simulink model "GSandFlare_werkend"  (R2021b)
settings: Solver=VariableStepAuto  StartTime=0.0  StopTime=140  RelTol=1e-3
values from neighbouring files (symbols this model uses):
  A_5 = SS_long_lo.A([1 2 3 4 5],[1 2 3 4 5])    [FindF16Dynamics.m]
  B_5 = SS_long_lo.A([1 2 3 4 5],[6 7])    [FindF16Dynamics.m]
  C_5 = SS_long_lo.C([1 2 3 4 5],[1 2 3 4 5])    [FindF16Dynamics.m]
  D_5 = SS_long_lo.D([1 2 3 4 5],[1 2])    [FindF16Dynamics.m]
  h_airport = 3000    [FindF16Dynamics.m]
  h_flare = x2*tan(GS_angle*(pi/180))    [FindF16Dynamics.m]
  runway_distance = 10*velocity + (2000/tan(GS_angle))    [FindF16Dynamics.m]
  tau = -h_flare/h_dot    [FindF16Dynamics.m]
  trim_alt = altitude    (= 5000)    [FindF16Dynamics.m]
  trim_velocity = velocity    (= 300)    [FindF16Dynamics.m]
undefined symbols (not defined in the file or in its folder): trim_state_lo, trim_thrust_lo
libraries: slpidlib x3
settings Model: Creator=Victor  LastModifiedBy=Victor

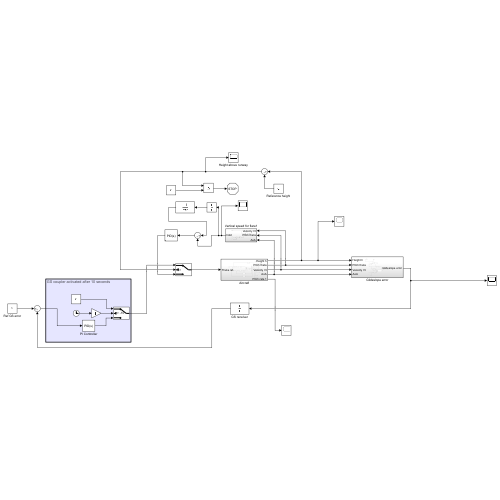
[thumbnail: Simulink's stored preview of the top-level diagram]
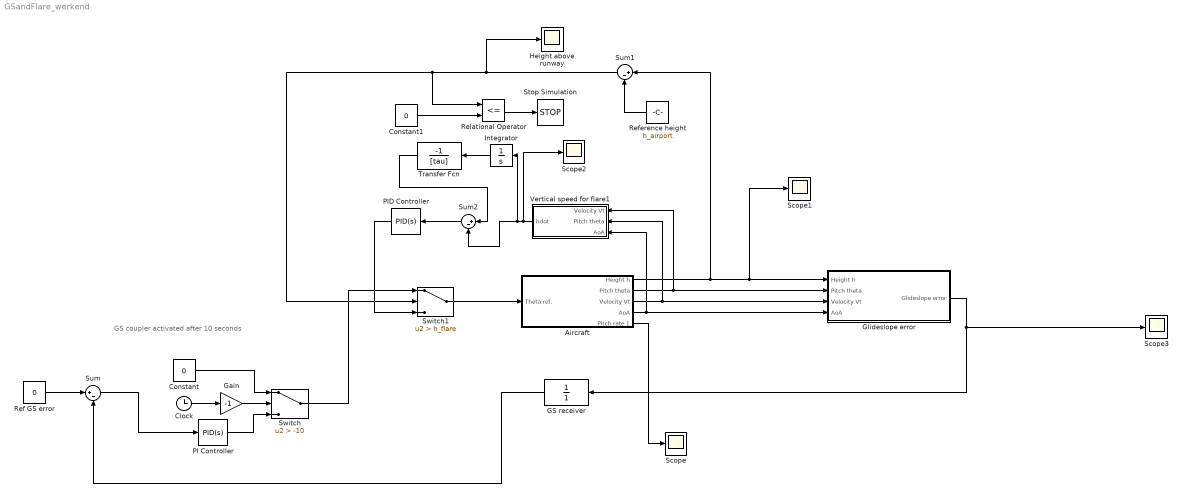
== system GSandFlare_werkend ==
  note: GS coupler activated after 10 seconds
  Aircraft : Subsystem  Tag=Aircraft
  Clock : Clock
  Constant : Constant  Value=0
  Constant1 : Constant  Value=0
  GS receiver : TransferFcn  Denominator=[1]
  Gain : Gain  Gain=-1
  Glideslope error : Subsystem
  Height above runway : Scope
  Integrator : Integrator
  PI Controller : slpidlib/PID Controller  Controller=PID  Form=Parallel  TimeDomain=Continuous-time  UseExternalTs=off  SampleTime=-1  IntegratorMethod=Forward Euler  FilterMethod=Forward Euler  ControllerParametersSource=internal  P=10  I=0.1  D=0  UseFilter=on  N=100  TunerSelectOption=Transfer Function Based (PID Tuner App)  InitialConditionSource=internal  InitialConditionForIntegrator=0  InitialConditionForFilter=0  DifferentiatorICPrevScaledInput=0  ExternalReset=none  TrackingMode=off  Kt=1  LimitOutput=off  SatLimitsSource=internal  UpperSaturationLimit=inf  LowerSaturationLimit=-inf  LinearizeAsGain=on  AntiWindupMode=none  Kb=1  POutMin=[]  POutMax=[]  IOutMin=[]  IOutMax=[]  DOutMin=[]  DOutMax=[]  NOutMin=[]  NOutMax=[]  SumOutMin=[]  SumOutMax=[]  SaturationOutMin=[]  SaturationOutMax=[]  PParamMin=[]  PParamMax=[]  IParamMin=[]  IParamMax=[]  DParamMin=[]  DParamMax=[]  NParamMin=[]  NParamMax=[]  KbParamMin=[]  KbParamMax=[]  KtParamMin=[]  KtParamMax=[]  KbOutMin=[]  KbOutMax=[]  KtOutMin=[]  KtOutMax=[]  IntegratorOutMin=[]  IntegratorOutMax=[]  FilterOutMin=[]  FilterOutMax=[]  SumI1OutMin=[]  SumI1OutMax=[]  SumI2OutMin=[]  SumI2OutMax=[]  SumI3OutMin=[]  SumI3OutMax=[]  SumI4OutMin=[]  SumI4OutMax=[]  SumDOutMin=[]  SumDOutMax=[]  DifferentiatorOutMin=[]  DifferentiatorOutMax=[]  FilterDiffOutCoefMin=[]  FilterDiffOutCoefMax=[]  ReciprocalOutMin=[]  ReciprocalOutMax=[]  SumDenOutMin=[]  SumDenOutMax=[]  SumNumOutMin=[]  SumNumOutMax=[]  DivideOutMin=[]  DivideOutMax=[]  UdiffTsProdOutMin=[]  UdiffTsProdOutMax=[]  NTsProdOutMin=[]  NTsProdOutMax=[]  UintegralTsProdOutMin=[]  UintegralTsProdOutMax=[]  UngainTsProdOutMin=[]  UngainTsProdOutMax=[]  IntegratorContinuousStateAttributes=''  IntegratorStateMustResolveToSignalObject=off  IntegratorRTWStateStorageClass=Auto  FilterContinuousStateAttributes=''  FilterStateMustResolveToSignalObject=off  FilterRTWStateStorageClass=Auto  ParallelPVariant=InternalParameters  IdealPVariant=Disabled  IVariant=InternalParameters  DVariant=InternalParameters  IntegratorVariant=Continuous  SatVariant=Disabled  AWVariant=Passthrough  PCopyVariant=Disabled  TRVariant=Disabled  FdbkBlocksVariant=Forward  IdealPFdbkVariant=Disabled  SatFdbkVariant=Disabled  DerivativeFilterVariant=ContFilter  NVariant=InternalParameters  NCopyVariant=Disabled  FilterICVariant=InternalICsFilter  IntegratorICVariant=InternalICs  ExternalResetVariant=Disabled  TRSumVariant=Passthrough  SumFdbkVariant=Disabled  SumVariant=Sum_PID  TsampFilterVariant=InternalTs  TsampNgainVariant=Passthrough  TsampIntegralVariant=Passthrough  ExternalSaturationOutDataTypeStr=Inherit: Same as second input
  PID Controller : slpidlib/PID Controller  Controller=PID  Form=Parallel  TimeDomain=Continuous-time  UseExternalTs=off  SampleTime=-1  IntegratorMethod=Forward Euler  FilterMethod=Forward Euler  ControllerParametersSource=internal  P=0.001  I=0.0000000001  D=0.45  UseFilter=on  N=100  TunerSelectOption=Transfer Function Based (PID Tuner App)  InitialConditionSource=internal  InitialConditionForIntegrator=0  InitialConditionForFilter=0  DifferentiatorICPrevScaledInput=0  ExternalReset=none  TrackingMode=off  Kt=1  LimitOutput=off  SatLimitsSource=internal  UpperSaturationLimit=inf  LowerSaturationLimit=-inf  LinearizeAsGain=on  AntiWindupMode=none  Kb=1  POutMin=[]  POutMax=[]  IOutMin=[]  IOutMax=[]  DOutMin=[]  DOutMax=[]  NOutMin=[]  NOutMax=[]  SumOutMin=[]  SumOutMax=[]  SaturationOutMin=[]  SaturationOutMax=[]  PParamMin=[]  PParamMax=[]  IParamMin=[]  IParamMax=[]  DParamMin=[]  DParamMax=[]  NParamMin=[]  NParamMax=[]  KbParamMin=[]  KbParamMax=[]  KtParamMin=[]  KtParamMax=[]  KbOutMin=[]  KbOutMax=[]  KtOutMin=[]  KtOutMax=[]  IntegratorOutMin=[]  IntegratorOutMax=[]  FilterOutMin=[]  FilterOutMax=[]  SumI1OutMin=[]  SumI1OutMax=[]  SumI2OutMin=[]  SumI2OutMax=[]  SumI3OutMin=[]  SumI3OutMax=[]  SumI4OutMin=[]  SumI4OutMax=[]  SumDOutMin=[]  SumDOutMax=[]  DifferentiatorOutMin=[]  DifferentiatorOutMax=[]  FilterDiffOutCoefMin=[]  FilterDiffOutCoefMax=[]  ReciprocalOutMin=[]  ReciprocalOutMax=[]  SumDenOutMin=[]  SumDenOutMax=[]  SumNumOutMin=[]  SumNumOutMax=[]  DivideOutMin=[]  DivideOutMax=[]  UdiffTsProdOutMin=[]  UdiffTsProdOutMax=[]  NTsProdOutMin=[]  NTsProdOutMax=[]  UintegralTsProdOutMin=[]  UintegralTsProdOutMax=[]  UngainTsProdOutMin=[]  UngainTsProdOutMax=[]  IntegratorContinuousStateAttributes=''  IntegratorStateMustResolveToSignalObject=off  IntegratorRTWStateStorageClass=Auto  FilterContinuousStateAttributes=''  FilterStateMustResolveToSignalObject=off  FilterRTWStateStorageClass=Auto  ParallelPVariant=InternalParameters  IdealPVariant=Disabled  IVariant=InternalParameters  DVariant=InternalParameters  IntegratorVariant=Continuous  SatVariant=Disabled  AWVariant=Passthrough  PCopyVariant=Disabled  TRVariant=Disabled  FdbkBlocksVariant=Forward  IdealPFdbkVariant=Disabled  SatFdbkVariant=Disabled  DerivativeFilterVariant=ContFilter  NVariant=InternalParameters  NCopyVariant=Disabled  FilterICVariant=InternalICsFilter  IntegratorICVariant=InternalICs  ExternalResetVariant=Disabled  TRSumVariant=Passthrough  SumFdbkVariant=Disabled  SumVariant=Sum_PID  TsampFilterVariant=InternalTs  TsampNgainVariant=Passthrough  TsampIntegralVariant=Passthrough  ExternalSaturationOutDataTypeStr=Inherit: Same as second input
  Ref GS error : Constant  Value=0
  Reference height : Constant  Value=h_airport
  Relational Operator : RelationalOperator  Operator=<=  OutDataTypeStr=boolean  RndMeth=Simplest
  Scope{,1..3} (4 alike) : Scope
  Stop Simulation : Stop
  Sum : Sum  Inputs=|+-
  Sum1 : Sum  Inputs=|+-
  Sum2 : Sum  Inputs=|+-
  Switch : Switch  Criteria=u2 > Threshold  Threshold=-10
  Switch1 : Switch  Criteria=u2 > Threshold  Threshold=h_flare
  Transfer Fcn : TransferFcn  Numerator=[-1]  Denominator=[tau]
  Vertical speed for flare1 : Subsystem
  wires:
  Aircraft/1(Height h) -> Sum1/1, Scope1/1, Glideslope error/1(Height h)
  Aircraft/4(AoA) -> Vertical speed for flare1/3(AoA), Glideslope error/4(AoA)
  Aircraft/2(Pitch theta) -> Vertical speed for flare1/1(Velocity Vt), Glideslope error/2(Pitch theta)
  Glideslope error/1(Glideslope error) -> GS receiver/1, Scope3/1
  Ref GS error/1 -> Sum/1
  GS receiver/1 -> Sum/2
  Sum/1 -> PI Controller/1
  PI Controller/1 -> Switch/3
  Constant/1 -> Switch/1
  Gain/1 -> Switch/2
  Clock/1 -> Gain/1
  Aircraft/3(Velocity Vt) -> Vertical speed for flare1/2(Pitch theta), Glideslope error/3(Velocity Vt)
  Switch/1 -> Switch1/1
  Switch1/1 -> Aircraft/1(Theta ref.)
  Reference height/1 -> Sum1/2
  Sum1/1 -> Height above runway/1, Relational Operator/1, Switch1/2
  Constant1/1 -> Relational Operator/2
  Relational Operator/1 -> Stop Simulation/1
  Aircraft/5(Pitch rate 1) -> Scope/1
  PID Controller/1 -> Switch1/3
  Vertical speed for flare1/1(hdot) -> Scope2/1, Integrator/1, Sum2/2
  Sum2/1 -> PID Controller/1
  Integrator/1 -> Transfer Fcn/1
  Transfer Fcn/1 -> Sum2/1

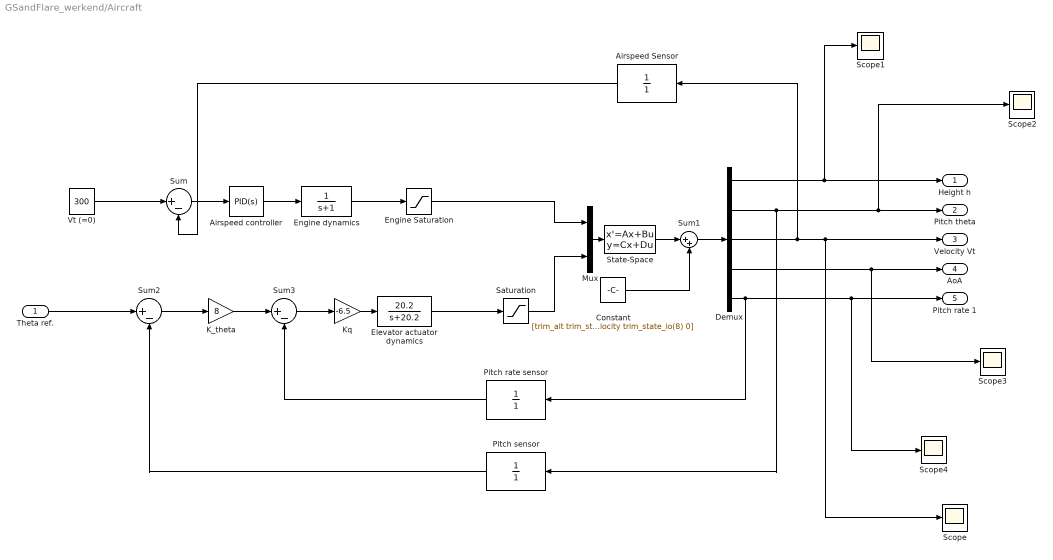
== system GSandFlare_werkend/Aircraft ==
  Theta ref. : Inport
  Airspeed Sensor : TransferFcn  Denominator=[1]
  Airspeed controller : slpidlib/PID Controller  Controller=PID  Form=Parallel  TimeDomain=Continuous-time  UseExternalTs=off  SampleTime=-1  IntegratorMethod=Forward Euler  FilterMethod=Forward Euler  ControllerParametersSource=internal  P=133.541176016203  I=2.35764233778221  D=232.681071797148  UseFilter=on  N=21.8595644116061  TunerSelectOption=Transfer Function Based (PID Tuner App)  InitialConditionSource=internal  InitialConditionForIntegrator=0  InitialConditionForFilter=0  DifferentiatorICPrevScaledInput=0  ExternalReset=none  TrackingMode=off  Kt=1  LimitOutput=off  SatLimitsSource=internal  UpperSaturationLimit=inf  LowerSaturationLimit=-inf  LinearizeAsGain=on  AntiWindupMode=none  Kb=1  POutMin=[]  POutMax=[]  IOutMin=[]  IOutMax=[]  DOutMin=[]  DOutMax=[]  NOutMin=[]  NOutMax=[]  SumOutMin=[]  SumOutMax=[]  SaturationOutMin=[]  SaturationOutMax=[]  PParamMin=[]  PParamMax=[]  IParamMin=[]  IParamMax=[]  DParamMin=[]  DParamMax=[]  NParamMin=[]  NParamMax=[]  KbParamMin=[]  KbParamMax=[]  KtParamMin=[]  KtParamMax=[]  KbOutMin=[]  KbOutMax=[]  KtOutMin=[]  KtOutMax=[]  IntegratorOutMin=[]  IntegratorOutMax=[]  FilterOutMin=[]  FilterOutMax=[]  SumI1OutMin=[]  SumI1OutMax=[]  SumI2OutMin=[]  SumI2OutMax=[]  SumI3OutMin=[]  SumI3OutMax=[]  SumI4OutMin=[]  SumI4OutMax=[]  SumDOutMin=[]  SumDOutMax=[]  DifferentiatorOutMin=[]  DifferentiatorOutMax=[]  FilterDiffOutCoefMin=[]  FilterDiffOutCoefMax=[]  ReciprocalOutMin=[]  ReciprocalOutMax=[]  SumDenOutMin=[]  SumDenOutMax=[]  SumNumOutMin=[]  SumNumOutMax=[]  DivideOutMin=[]  DivideOutMax=[]  UdiffTsProdOutMin=[]  UdiffTsProdOutMax=[]  NTsProdOutMin=[]  NTsProdOutMax=[]  UintegralTsProdOutMin=[]  UintegralTsProdOutMax=[]  UngainTsProdOutMin=[]  UngainTsProdOutMax=[]  IntegratorContinuousStateAttributes=''  IntegratorStateMustResolveToSignalObject=off  IntegratorRTWStateStorageClass=Auto  FilterContinuousStateAttributes=''  FilterStateMustResolveToSignalObject=off  FilterRTWStateStorageClass=Auto  ParallelPVariant=InternalParameters  IdealPVariant=Disabled  IVariant=InternalParameters  DVariant=InternalParameters  IntegratorVariant=Continuous  SatVariant=Disabled  AWVariant=Passthrough  PCopyVariant=Disabled  TRVariant=Disabled  FdbkBlocksVariant=Forward  IdealPFdbkVariant=Disabled  SatFdbkVariant=Disabled  DerivativeFilterVariant=ContFilter  NVariant=InternalParameters  NCopyVariant=Disabled  FilterICVariant=InternalICsFilter  IntegratorICVariant=InternalICs  ExternalResetVariant=Disabled  TRSumVariant=Passthrough  SumFdbkVariant=Disabled  SumVariant=Sum_PID  TsampFilterVariant=InternalTs  TsampNgainVariant=Passthrough  TsampIntegralVariant=Passthrough  ExternalSaturationOutDataTypeStr=Inherit: Same as second input
  Constant : Constant  Value=[trim_alt trim_state_lo(5) trim_velocity trim_state_lo(8) 0]
  Demux : Demux  Outputs=5
  Elevator actuator dynamics : TransferFcn  Numerator=[20.2]  Denominator=[1 20.2]
  Engine Saturation : Saturate  UpperLimit=19000 -trim_thrust_lo  LowerLimit=1000 - trim_thrust_lo
  Engine dynamics : TransferFcn  Denominator=[1 1]
  K_theta : Gain  Gain=8
  Kq : Gain  Gain=-6.5
  Mux : Mux  Inputs=2
  Pitch rate sensor : TransferFcn  Denominator=[1]
  Pitch sensor : TransferFcn  Denominator=[1]
  Saturation : Saturate  UpperLimit=25  LowerLimit=-25
  Scope{,1..4} (5 alike) : Scope
  State-Space : StateSpace  A=A_5  B=B_5  C=C_5  D=D_5  InitialCondition=0  ParameterTunability=Unconstrained
  Sum : Sum  Inputs=|+-
  Sum1 : Sum  Inputs=|++
  Sum2 : Sum  Inputs=|+-
  Sum3 : Sum  Inputs=|+-
  Vt (=0) : Constant  Value=300
  Height h : Outport
  Pitch theta : Outport  Port=2
  Velocity Vt : Outport  Port=3
  AoA : Outport  Port=4
  Pitch rate 1 : Outport  Port=5
  wires:
  Demux/1 -> Scope1/1, Height h/1
  Demux/2 -> Pitch sensor/1, Scope2/1, Pitch theta/1
  Demux/4 -> Scope3/1, AoA/1
  Demux/5 -> Scope4/1, Pitch rate 1/1, Pitch rate sensor/1
  Vt (=0)/1 -> Sum/1
  Airspeed Sensor/1 -> Sum/2
  Sum/1 -> Airspeed controller/1
  Airspeed controller/1 -> Engine dynamics/1
  Engine dynamics/1 -> Engine Saturation/1
  Mux/1 -> State-Space/1
  Engine Saturation/1 -> Mux/1
  Theta ref./1 -> Sum2/1
  Sum2/1 -> K_theta/1
  K_theta/1 -> Sum3/1
  Sum3/1 -> Kq/1
  Kq/1 -> Elevator actuator dynamics/1
  Pitch rate sensor/1 -> Sum3/2
  Pitch sensor/1 -> Sum2/2
  Demux/3 -> Airspeed Sensor/1, Scope/1, Velocity Vt/1
  Saturation/1 -> Mux/2
  State-Space/1 -> Sum1/1
  Sum1/1 -> Demux/1
  Constant/1 -> Sum1/2
  Elevator actuator dynamics/1 -> Saturation/1

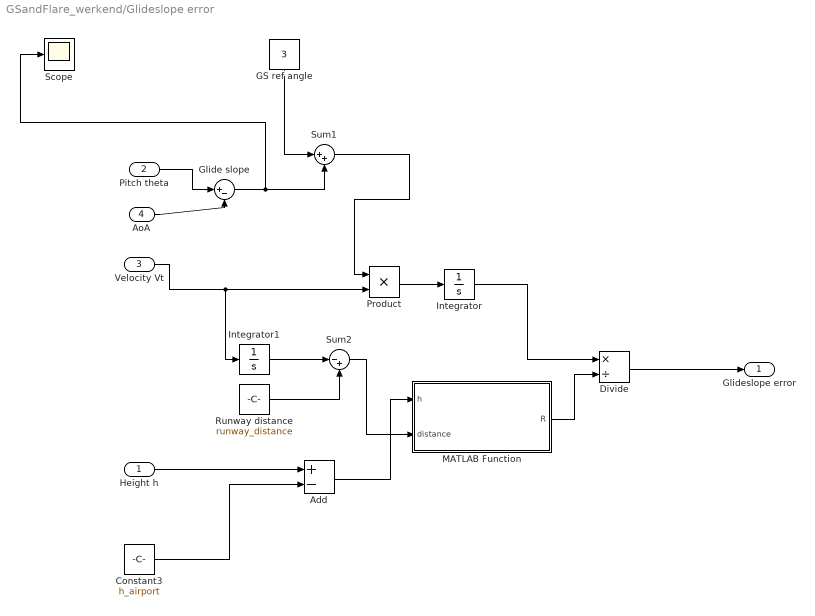
== system GSandFlare_werkend/Glideslope error ==
  Height h : Inport
  Pitch theta : Inport  Port=2
  Velocity Vt : Inport  Port=3
  AoA : Inport  Port=4
  Add : Sum  Inputs=+-
  Constant3 : Constant  Value=h_airport
  Divide : Product  Inputs=*/
  GS ref angle : Constant  Value=3
  Glide slope : Sum  Inputs=|+-
  Integrator : Integrator
  Integrator1 : Integrator
  MATLAB Function : MATLAB Function  TreatAsAtomicUnit=on
  Product : Product
  Runway distance : Constant  Value=runway_distance
  Scope : Scope
  Sum1 : Sum  Inputs=|++
  Sum2 : Sum  Inputs=|-+
  Glideslope error : Outport
  wires:
  AoA/1 -> Glide slope/2
  Pitch theta/1 -> Glide slope/1
  Glide slope/1 -> Scope/1, Sum1/2
  GS ref angle/1 -> Sum1/1
  Sum1/1 -> Product/1
  Velocity Vt/1 -> Integrator1/1, Product/2
  Product/1 -> Integrator/1
  Integrator/1 -> Divide/1
  Height h/1 -> Add/1
  Runway distance/1 -> Sum2/2
  Integrator1/1 -> Sum2/1
  Add/1 -> MATLAB Function/1(h)
  Sum2/1 -> MATLAB Function/2(distance)
  MATLAB Function/1(R) -> Divide/2
  Divide/1 -> Glideslope error/1
  Constant3/1 -> Add/2

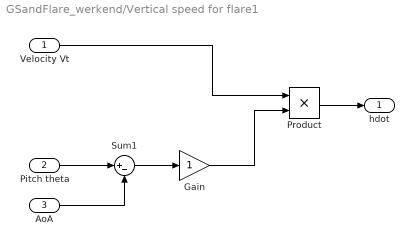
== system GSandFlare_werkend/Vertical speed for flare1 ==
  Velocity Vt : Inport
  Pitch theta : Inport  Port=2
  AoA : Inport  Port=3
  Gain : Gain
  Product : Product
  Sum1 : Sum  Inputs=|+-
  hdot : Outport
  wires:
  Pitch theta/1 -> Sum1/1
  AoA/1 -> Sum1/2
  Velocity Vt/1 -> Product/1
  Sum1/1 -> Gain/1
  Product/1 -> hdot/1
  Gain/1 -> Product/2

== matlab function GSandFlare_werkend/Glideslope error/MATLAB Function ==
  data: R output; h input; distance input
function R = fcn(h,distance)

R = sqrt(h^2 + distance^2);
